simulink model "Mdl_12_CloseLoop_dn"  (R2018a)
settings: Solver=VariableStepAuto  StartTime=0.0  StopTime=10.0  RelTol=1e-3
undefined symbols (not defined in the file): A_mdl, B_mdl, C_mdl, D_mdl, K_d_mdl, Ts
settings Model: Creator=pala  LastModifiedBy=pala
settings DataIOCC: FinalStateName=xF_CL_dn  SaveFinalState=on  SaveFormat=StructureWithTime  SaveState=on  SignalLogging=off  DSMLogging=off  StateSaveName=x_CL_dn  TimeSaveName=t_CL_dn  OutputSaveName=y_CL_dn

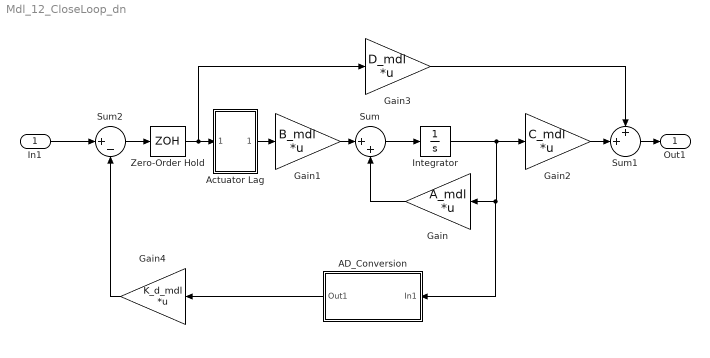
== system Mdl_12_CloseLoop_dn ==
  In1 : Inport  PortDimensions=2
  AD_Conversion : Subsystem
  Actuator Lag : Subsystem
  Gain : Gain  Gain=A_mdl  Multiplication=Matrix(K*u)
  Gain1 : Gain  Gain=B_mdl  Multiplication=Matrix(K*u)
  Gain2 : Gain  Gain=C_mdl  Multiplication=Matrix(K*u)
  Gain3 : Gain  Gain=D_mdl  Multiplication=Matrix(K*u)
  Gain4 : Gain  Gain=K_d_mdl  Multiplication=Matrix(K*u)
  Integrator : Integrator
  Sum : Sum  Inputs=|++
  Sum1 : Sum  Inputs=++|
  Sum2 : Sum  Inputs=|+-
  Zero-Order Hold : ZeroOrderHold  SampleTime=Ts
  Out1 : Outport
  wires:
  Gain/1 -> Sum/2
  Sum/1 -> Integrator/1
  Integrator/1 -> Gain2/1, AD_Conversion/1(In1), Gain/1
  Gain1/1 -> Sum/1
  Gain2/1 -> Sum1/2
  Sum1/1 -> Out1/1
  Gain3/1 -> Sum1/1
  In1/1 -> Sum2/1
  Sum2/1 -> Zero-Order Hold/1
  Gain4/1 -> Sum2/2
  AD_Conversion/1(Out1) -> Gain4/1
  Zero-Order Hold/1 -> Gain3/1, Actuator Lag/1(In1)
  Actuator Lag/1(Out1) -> Gain1/1

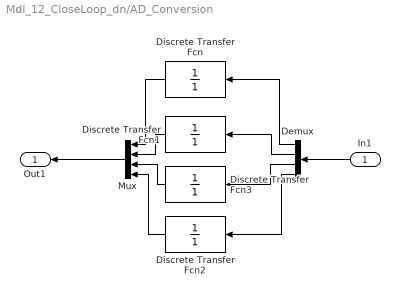
== system Mdl_12_CloseLoop_dn/AD_Conversion ==
  In1 : Inport
  Demux : Demux
  Discrete Transfer Fcn{,1..3} (4 alike) : DiscreteTransferFcn  Denominator=[1]  SampleTime=Ts
  Mux : Mux
  Out1 : Outport
  wires:
  Discrete Transfer Fcn2/1 -> Mux/4
  Demux/4 -> Discrete Transfer Fcn2/1
  Demux/3 -> Discrete Transfer Fcn3/1
  In1/1 -> Demux/1
  Discrete Transfer Fcn3/1 -> Mux/3
  Discrete Transfer Fcn/1 -> Mux/1
  Mux/1 -> Out1/1
  Discrete Transfer Fcn1/1 -> Mux/2
  Demux/1 -> Discrete Transfer Fcn/1
  Demux/2 -> Discrete Transfer Fcn1/1

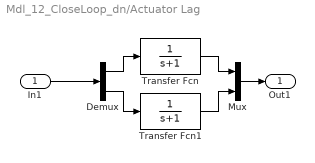
== system Mdl_12_CloseLoop_dn/Actuator Lag ==
  In1 : Inport
  Demux : Demux  Outputs=2
  Mux : Mux  Inputs=2
  Transfer Fcn : TransferFcn  Denominator=[1 1]
  Transfer Fcn1 : TransferFcn  Denominator=[1 1]
  Out1 : Outport
  wires:
  Demux/1 -> Transfer Fcn/1
  Demux/2 -> Transfer Fcn1/1
  In1/1 -> Demux/1
  Mux/1 -> Out1/1
  Transfer Fcn/1 -> Mux/1
  Transfer Fcn1/1 -> Mux/2
